simulink model "fuzzypid"  (R2022b)
settings: Solver=VariableStepAuto  StartTime=0.0  StopTime=50.0  RelTol=1e-3
libraries: fuzblock x2
settings Model: Creator=HP  LastModifiedBy=HP

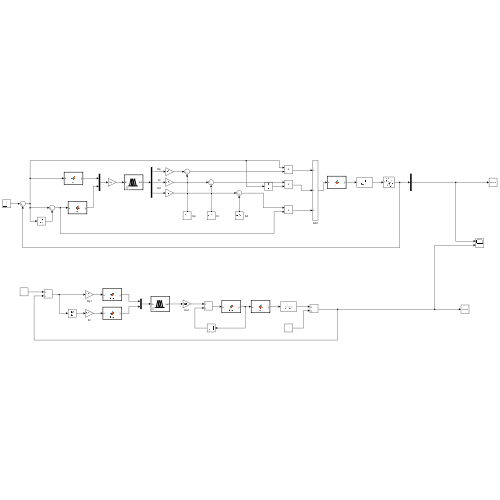
[thumbnail: Simulink's stored preview of the top-level diagram]
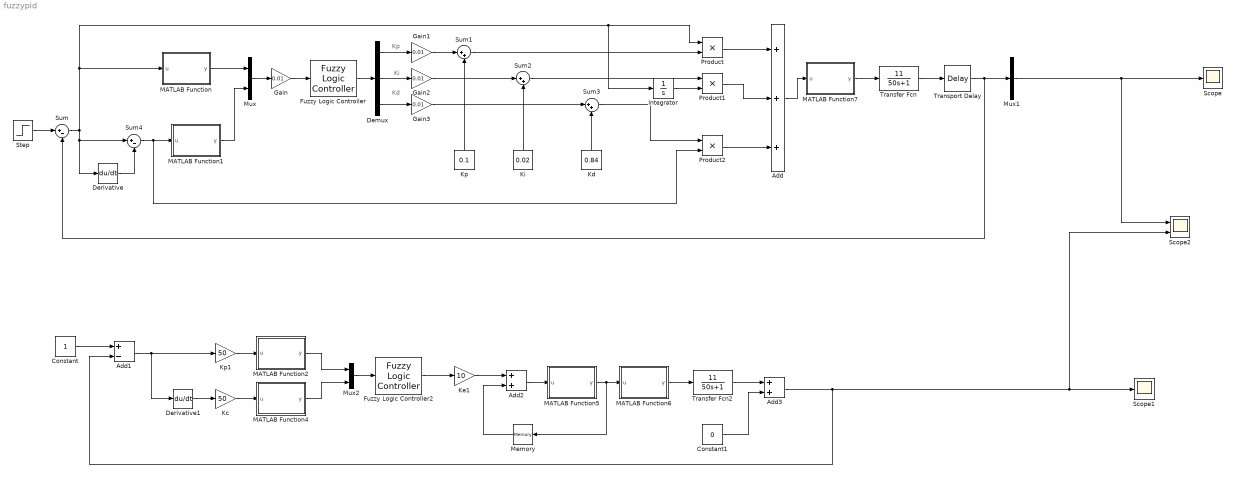
== system fuzzypid ==
  note: Kp
  note: Ki
  note: Kd
  Add : Sum  Inputs=+++
  Add1 : Sum  Inputs=+-
  Add2 : Sum
  Add3 : Sum
  Constant : Constant
  Constant1 : Constant  Value=0
  Demux : Demux  Outputs=3
  Derivative : Derivative
  Derivative1 : Derivative
  Fuzzy Logic Controller : fuzblock/Fuzzy Logic  Controller  FIS='fuzzypid.fis'  OutputSampleNumber=101  DataType=double  FuzzifiedInputs=off  RuleFiringStrengths=off  RuleOutputs=off  AggregatedOutputs=off  SimulateUsing=Interpreted execution  OutOfRangeInputValueMessage=warning  NoRuleFiredMessage=warning  EmptyOutputFuzzySetMessage=warning
  Fuzzy Logic Controller2 : fuzblock/Fuzzy Logic  Controller  FIS='fuzzytry.fis'  OutputSampleNumber=101  DataType=double  FuzzifiedInputs=off  RuleFiringStrengths=off  RuleOutputs=off  AggregatedOutputs=off  SimulateUsing=Interpreted execution  OutOfRangeInputValueMessage=warning  NoRuleFiredMessage=warning  EmptyOutputFuzzySetMessage=warning
  Gain{,1..3} (4 alike) : Gain  Gain=0.01
  Integrator : Integrator
  Kc : Gain  Gain=50
  Kd : Constant  Value=0.84
  Ke1 : Gain  Gain=10
  Ki : Constant  Value=0.02
  Kp : Constant  Value=0.1
  Kp1 : Gain  Gain=50
  MATLAB Function : MATLAB Function  TreatAsAtomicUnit=on
  MATLAB Function1 : MATLAB Function  TreatAsAtomicUnit=on
  MATLAB Function2 : MATLAB Function  TreatAsAtomicUnit=on
  MATLAB Function4 : MATLAB Function  TreatAsAtomicUnit=on
  MATLAB Function5 : MATLAB Function  TreatAsAtomicUnit=on
  MATLAB Function6 : MATLAB Function  TreatAsAtomicUnit=on
  MATLAB Function7 : MATLAB Function  TreatAsAtomicUnit=on
  Memory : Memory
  Mux : Mux  Inputs=2
  Mux1 : Mux  Inputs=1
  Mux2 : Mux  Inputs=2
  Product : Product
  Product1 : Product
  Product2 : Product
  Scope : Scope
  Scope1 : Scope
  Scope2 : Scope  NumInputPorts=2
  Step : Step  SampleTime=0
  Sum : Sum  Inputs=|+-
  Sum1 : Sum  Inputs=|++
  Sum2 : Sum  Inputs=|++
  Sum3 : Sum  Inputs=|++
  Sum4 : Sum  Inputs=|+-
  Transfer Fcn : TransferFcn  Numerator=[11]  Denominator=[50 1]
  Transfer Fcn2 : TransferFcn  Numerator=[11]  Denominator=[50 1]
  Transport Delay : TransportDelay
  wires:
  Step/1 -> Sum/1
  Sum/1 -> Sum4/1, Derivative/1, Integrator/1, Product/1, MATLAB Function/1(u)
  Mux/1 -> Gain/1
  Fuzzy Logic Controller/1 -> Demux/1
  Demux/3 -> Gain3/1
  Demux/1 -> Gain1/1
  Transfer Fcn/1 -> Transport Delay/1
  Transport Delay/1 -> Mux1/1, Sum/2
  Gain/1 -> Fuzzy Logic Controller/1
  Demux/2 -> Gain2/1
  Kp/1 -> Sum1/2
  Gain1/1 -> Sum1/1
  Gain2/1 -> Sum2/1
  Ki/1 -> Sum2/2
  Gain3/1 -> Sum3/1
  Kd/1 -> Sum3/2
  Sum1/1 -> Product/2
  Product/1 -> Add/1
  Sum2/1 -> Product1/1
  Integrator/1 -> Product1/2
  Product1/1 -> Add/2
  Sum3/1 -> Product2/1
  Product2/1 -> Add/3
  Mux1/1 -> Scope2/1, Scope/1
  MATLAB Function/1(y) -> Mux/1
  MATLAB Function1/1(y) -> Mux/2
  Add/1 -> MATLAB Function7/1(u)
  Derivative1/1 -> Kc/1
  Transfer Fcn2/1 -> Add3/1
  Add2/1 -> MATLAB Function5/1(u)
  MATLAB Function4/1(y) -> Mux2/2
  Add1/1 -> Derivative1/1, Kp1/1
  MATLAB Function5/1(y) -> Memory/1, MATLAB Function6/1(u)
  Kc/1 -> MATLAB Function4/1(u)
  Fuzzy Logic Controller2/1 -> Ke1/1
  Kp1/1 -> MATLAB Function2/1(u)
  MATLAB Function2/1(y) -> Mux2/1
  Add3/1 -> Add1/2, Scope2/2, Scope1/1
  Constant/1 -> Add1/1
  Mux2/1 -> Fuzzy Logic Controller2/1
  MATLAB Function6/1(y) -> Transfer Fcn2/1
  Constant1/1 -> Add3/2
  Ke1/1 -> Add2/1
  Memory/1 -> Add2/2
  MATLAB Function7/1(y) -> Transfer Fcn/1
  Derivative/1 -> Sum4/2
  Sum4/1 -> Product2/2, MATLAB Function1/1(u)

== matlab function fuzzypid/MATLAB Function ==
  data: u input; y output
function y = fcn(u)
vmax = 6;
vmin = -6;
if u > vmax
    u = vmax;
end
if u < vmin
    u = vmin;
end
y = u;

== matlab function fuzzypid/MATLAB Function2 ==
  data: u input; y output
function y = fcn(u)
vmax = 6;
vmin = -6;
if u > vmax
    u = vmax;
end
if u < vmin
    u = vmin;
end
y = u;

== matlab function fuzzypid/MATLAB Function4 ==
  data: u input; y output
function y = fcn(u)
vmax = 6;
vmin = -6;
if u > vmax
    u = vmax;
end
if u < vmin
    u = vmin;
end
y = u;

== matlab function fuzzypid/MATLAB Function5 ==
  data: u input; y output
function y = fcn(u)
vmax = 1;
vmin = -1;
if u > vmax
    u = vmax;
end
if u < vmin
    u = vmin;
end
y = u;

== matlab function fuzzypid/MATLAB Function6 ==
  data: u input; y output
function y = fcn(u)
vmax = 1;
vmin = 0;
if u > vmax
    u = vmax;
end
if u < vmin
    u = vmin;
end
y = u;

== matlab function fuzzypid/MATLAB Function7 ==
  data: u input; y output
function y = fcn(u)
vmax = 1;
vmin = 0;
if u > vmax
    u = vmax;
end
if u < vmin
    u = vmin;
end
y = u;

== matlab function fuzzypid/MATLAB Function1 ==
  data: u input; y output
function y = fcn(u)
vmax = 6;
vmin = -6;
if u > vmax
    u = vmax;
end
if u < vmin
    u = vmin;
end
y = u;
